simulink model "penduloSLX"  (R2020b)
settings: Solver=VariableStepAuto  StartTime=0.0  StopTime=10.0  RelTol=1e-3
values from neighbouring files (symbols this model uses):
  y0 = [1 0]'    [DSF_TP0_S24.m]    (also in DSF_TP0_S31_FIXED.m; DSF_TP0_S32_ODE15s.m; DSF_TP0_S32_ODE45.m; DSF_TP0_S32_ODE45_DECIMADO.m)
settings Model: Creator=luis  LastModifiedBy=luis

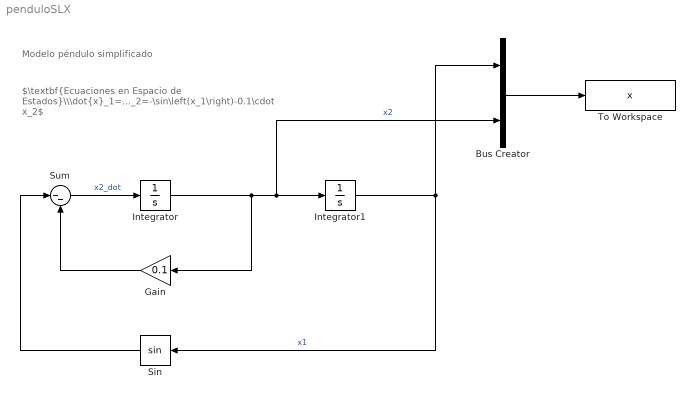
== system penduloSLX ==
  note: Modelo péndulo simplificado
  note: $\textbf{Ecuaciones en Espacio de Estados}\\\dot{x}_1=x_2\\\dot{x}_2=-\sin\left(x_1\right)-0.1\cdot x_2$
  Bus Creator : BusCreator  Inputs=2
  Gain : Gain  Gain=0.1
  Integrator : Integrator  InitialCondition=y0(2)
  Integrator1 : Integrator  InitialCondition=y0(1)
  Sin : Trigonometry
  Sum : Sum  Inputs=|--
  To Workspace : ToWorkspace  VariableName=x  SaveFormat=Timeseries  SampleTime=-1
  wires:
  Integrator/1 -> Gain/1, Bus Creator/2, Integrator1/1  "x2"
  Sum/1 -> Integrator/1  "x2_dot"
  Integrator1/1 -> Bus Creator/1, Sin/1  "x1"
  Gain/1 -> Sum/2
  Sin/1 -> Sum/1
  Bus Creator/1 -> To Workspace/1
